simulink model "M_ZH_Z2"  (R2025a)
settings: Solver=VariableStepAuto  StartTime=0.0  StopTime=25  MaxStep=100e-3  RelTol=1e-3
settings Model: Creator=Szalay  LastModifiedBy=Szalay

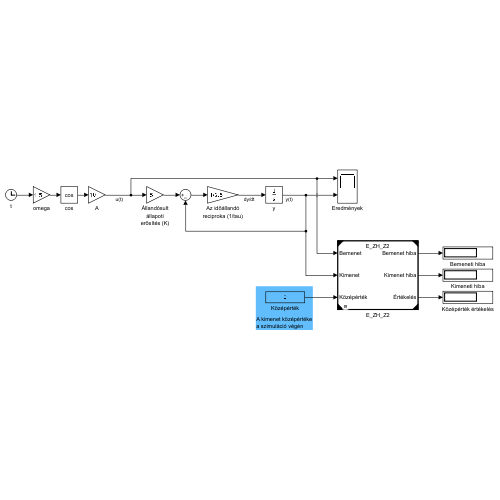
[thumbnail: Simulink's stored preview of the top-level diagram]
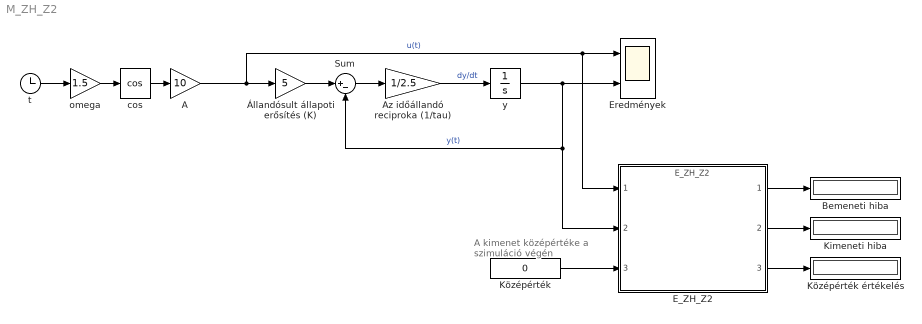
== system M_ZH_Z2 ==
  note: A kimenet középértéke
      | a szimuláció végén
  A : Gain  Gain=10
  Az időállandó reciproka (1/tau) : Gain  Gain=1/2.5
  Bemeneti hiba : Display
  E_ZH_Z2 : ModelReference  ModelNameDialog=E_ZH_Z2.slxp  ModelReferenceVersion=1.14  CopyOfModelProtected=on
  Eredmények : Scope  NumInputPorts=2
      settings: ActiveDisplayYMinimum=-12.499602407802596  ActiveDisplayYMaximum=12.499955823089177
  Kimeneti hiba : Display
  Középérték : Constant  Value=0
  Középérték értékelés : Display
  Sum : Sum  Inputs=|+-
  cos : Trigonometry  Operator=cos
  omega : Gain  Gain=1.5
  t : Clock
  y : Integrator  InitialCondition=-20
  Állandósult állapoti erősítés (K) : Gain  Gain=5
  wires:
  t/1 -> omega/1
  cos/1 -> A/1
  A/1 -> E_ZH_Z2/1, Eredmények/1, Állandósult állapoti erősítés (K)/1  "u(t)"
  Állandósult állapoti erősítés (K)/1 -> Sum/1
  Sum/1 -> Az időállandó reciproka (1/tau)/1
  Az időállandó reciproka (1/tau)/1 -> y/1  "dy/dt"
  y/1 -> E_ZH_Z2/2, Sum/2, Eredmények/2  "y(t)"
  E_ZH_Z2/1 -> Bemeneti hiba/1
  E_ZH_Z2/2 -> Kimeneti hiba/1
  omega/1 -> cos/1
  E_ZH_Z2/3 -> Középérték értékelés/1
  Középérték/1 -> E_ZH_Z2/3
